simulink model "ModelForPicture"  (R2023a)
settings: Solver=VariableStepAuto  StartTime=0.0  StopTime=10.0  RelTol=1e-3
values from neighbouring files (symbols this model uses):
  timeStep = 0.005    [Cosim_Setup_SLC_MPC_T1_SP_LTR_Cosim_3D.m]
libraries: simulink x7, Solver_SF x1
settings Model: Creator=28303  LastModifiedBy=28303

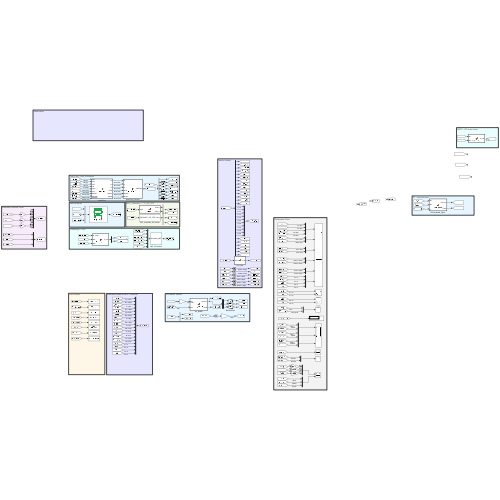
[thumbnail: Simulink's stored preview of the top-level diagram]
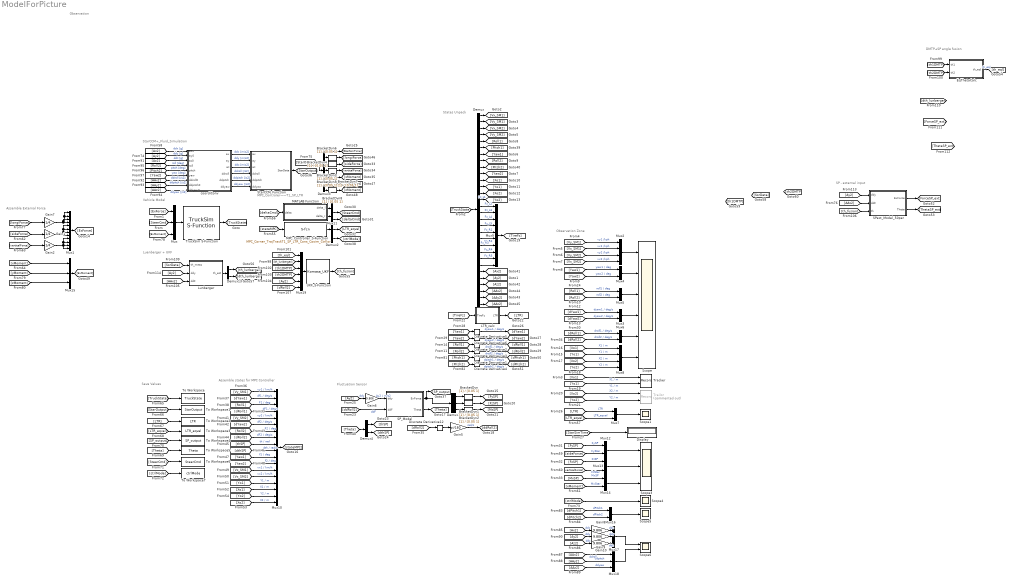
== system ModelForPicture ==
  note: Save Values
  note: StarCCM+_Fluid_Simulation
  note: Assemble states for MPC Controller
  note: Observation Zone
  note: Vehicle Model
  note: Fluctuation Sensor
  note: States Unpack
  note: Assemble External Force
  note: MPC_Controler——T1_SP_LTR
  note: Observation
  note: Luenberger + UKF
  note: SP - external input
  note: DMTP→SP angle fusion
  BracketDyn{,1..8} (9 alike) : TransferFcn  Denominator=[0.05 1]
  Demux : Demux  Outputs=30
  Demux1 : Demux  Outputs=3
  Demux13 : Demux  Outputs=2
  Demux2 : Demux  Outputs=3
  Demux3 : Demux  Outputs=7
  Demux4 : Demux  Outputs=2
  Discrete Derivative{1..6,12} (7 alike) : simulink/Discrete/Discrete Derivative  gainval=1.0  ICPrevScaledInput=0.0  OutMin=[]  OutMax=[]  OutDataType=fixdt(1, 16)  OutScaling=2^-10  DoSatur=off
  Display : Display
  EqThetaCalc : MATLAB Function  TreatAsAtomicUnit=on
  Gain1 : Gain  Gain=1/4
  Gain{6,8..10} (4 alike) : Gain  Gain=9.806
  Gain2 : Gain  Gain=1/4
  Gain5 : Gain  Gain=pi/180
  Gain7 : Gain  Gain=1/4
  "LTR_calc " : MATLAB Function  TreatAsAtomicUnit=on
  Lunberger : MATLAB Function  TreatAsAtomicUnit=on  SystemSampleTime=0.005
  MATLAB Function : MATLAB Function  TreatAsAtomicUnit=on
  MPC_Controller_S-Function : S-Function  FunctionName=MPC_Corner_TrajTrackT1_SP_LTR_Cons_Cosim_Ctrllor  SFunctionDeploymentMode=off  EnableBusSupport=off
  Mux{,15,17..18} (4 alike) : Mux  Inputs=3
  Mux1 : Mux  Inputs=12
  Mux10 : Mux  Inputs=18
  Mux{3..7,11..14,16} (10 alike) : Mux  Inputs=2
  Mux19 : Mux  Inputs=6
  Mux2 : Mux
  Mux8 : Mux
  Mux9 : Mux  Inputs=10
  SP_Model : MATLAB Function  TreatAsAtomicUnit=on  SystemSampleTime=0.005
  SPext_Model_50per : MATLAB Function  TreatAsAtomicUnit=on  SystemSampleTime=0.005
  Scope : Scope  NumInputPorts=6
  Scope1 : Scope
  Scope3 : Scope  NumInputPorts=3
  Scope4 : Scope
  Scope5 : Scope
  Scope6 : Scope  NumInputPorts=2
  StarCCM_Function : MATLAB Function  TreatAsAtomicUnit=on  SystemSampleTime=[timeStep 0]
  To Workspace : ToWorkspace  VariableName=TruckState  SaveFormat=Timeseries  SampleTime=-1
  To Workspace1 : ToWorkspace  VariableName=StarOutput  SaveFormat=Timeseries  SampleTime=-1
  To Workspace2 : ToWorkspace  VariableName=LTR  SaveFormat=Timeseries  SampleTime=-1
  To Workspace3 : ToWorkspace  VariableName=LTR_eqval  SaveFormat=Timeseries  SampleTime=-1
  To Workspace4 : ToWorkspace  VariableName=SP_output  SaveFormat=Timeseries  SampleTime=-1
  To Workspace5 : ToWorkspace  VariableName=Theta  SaveFormat=Timeseries  SampleTime=-1
  To Workspace6 : ToWorkspace  VariableName=SteerCmd  SaveFormat=Timeseries  SampleTime=-1
  To Workspace7 : ToWorkspace  VariableName=ctrlMode  SaveFormat=Timeseries  SampleTime=-1
  Tracker : Record  FileSettingsInternal="{\"entries\":[{\"content\":{\"excelSettings\":{\"content\":{},\"type\":\"Streamout.ExcelSettings\"}},\"type\":\"Streamout.FileSettingStorage\",\"uuid\":\"4a90c35d-7bfd-41ec-8da0-5aca52dec46b\"}],\"packageUris\":[\"http://schema.mathworks.com/mf0/streamout_blocks/R2020a\"],\"version\":\"1.0\"}"  Layout=[1 1]  SignalsInternal="{\"entries\":[{\"content\":{\"signals\":[{\"content\":{\"blockPath\":[\"ModelForPicture/Tracker\"],\"dimensions\":[1],\"domain\":\"ModelForPicture/Tracker\",\"lineColor\":\"#a2142f\",\"plots\":[1],\"port\":1,\"signalID\":60,\"signalName\":\"X1 / m\"},\"type\":\"RecordBlkView.Signal\",\"uuid\":\"e0ec3f2a-d673-4e95-a2c3-a892657a70bc\"},{\"content\":{\"blockPath\":[\"ModelForPicture/Tracker\"],\"dimensions\":[1],\"domain\":\"ModelForPicture/Tracker\",\"lineColor\":\"#139fff\",\"plots\":[1],\"port\":2,\"signalID\":63,\"signalName\":\"Y1 / m\"},\"type\":\"RecordBlkView.Signal\",\"uuid\":\"7fecea9c-d846-4e34-85a3-bedaa984d42a\"}]},\"type\":\"RecordBlkView.InputSignals\",\"uuid\":\"c903ce25-8e67-4217-b729-18382a9d9747\"}],\"packageUris\":[\"http://schema.mathworks.com/mf0/streamout_blocks/R2020a\"],\"version\":\"1.0\"}"  VisualizationBindings="{\"xyplotplugin\":{\"info\":[{\"series\":[{\"bindingParametersList\":[{\"parameter\":\"X-Axis\",\"signalID\":60,\"signalName\":\"X1 \\/ m\"},{\"parameter\":\"Y-Axis\",\"signalID\":63,\"signalName\":\"Y1 \\/ m\"}],\"seriesID\":59350}],\"subplotID\":1}]}}"  CompatibilityTag=XY  st=-1
  "Trailor " : Record  Commented=on  FileSettingsInternal="{\"entries\":[{\"content\":{\"excelSettings\":{\"content\":{},\"type\":\"Streamout.ExcelSettings\"}},\"type\":\"Streamout.FileSettingStorage\",\"uuid\":\"feb93b89-5eaa-4280-93fa-8b27e2285d0c\"}],\"packageUris\":[\"http://schema.mathworks.com/mf0/streamout_blocks/R2020a\"],\"version\":\"1.0\"}"  Layout=[1 1]  SignalsInternal="{\"entries\":[{\"content\":{\"signals\":[{\"content\":{\"blockPath\":[\"ModelForPicture/Trailor \"],\"dimensions\":[1],\"domain\":\"ModelForPicture/Trailor \",\"lineColor\":\"#a2142f\",\"plots\":[1],\"port\":1,\"signalID\":52,\"signalName\":\"XY Graph:1\"},\"type\":\"RecordBlkView.Signal\",\"uuid\":\"cce15bee-6aac-4d00-ab61-70a8d4efd641\"},{\"content\":{\"blockPath\":[\"ModelForPicture/Trailor \"],\"dimensions\":[1],\"domain\":\"ModelForPicture/Trailor \",\"lineColor\":\"#139fff\",\"plots\":[1],\"port\":2,\"signalID\":55,\"signalName\":\"XY Graph:2\"},\"type\":\"RecordBlkView.Signal\",\"uuid\":\"4f8b7c47-76ec-4c22-8b6d-3fa533720d48\"}]},\"type\":\"RecordBlkView.InputSignals\",\"uuid\":\"e5dfdc97-ae74-4c5b-8c00-5dfecc099489\"}],\"packageUris\":[\"http://schema.mathworks.com/mf0/streamout_blocks/R2020a\"],\"version\":\"1.0\"}"  VisualizationBindings="{\"xyplotplugin\":{\"info\":[{\"series\":[{\"bindingParametersList\":[{\"parameter\":\"X-Axis\",\"signalID\":52,\"signalName\":\"XY Graph:1\"},{\"parameter\":\"Y-Axis\",\"signalID\":55,\"signalName\":\"XY Graph:2\"}],\"seriesID\":41172}],\"subplotID\":1}]}}"  CompatibilityTag=XY  st=-1
  TruckSim S-Function : Solver_SF/TruckSim S-Function  Priority=1  SIMFILE=ALGO_Corner_Tanker_TrajTrack_MPC_T1_SP_LTR_Cosim_3D.sim
      settings: SourceProductName=TruckSim S-Function
  UKF_S-Function : S-Function  FunctionName=Komasa_UKF  SFunctionDeploymentMode=off  EnableBusSupport=off
  coordiConv : MATLAB Function  TreatAsAtomicUnit=on
  wires:
  Demux/23 -> Mux9/9  "Fz_R5"
  Demux2/3 -> [ctrlMode]
  [ctrlMode] -> To Workspace7/1
  [stateMPC] -> MPC_Controller_S-Function/1
  Demux/24 -> Mux9/10
  [Vx_SM2] -> Mux10/14  "vx2 / km/h"
  Mux12/1 -> Scope3/1
  [Yaw1] -> Mux10/11  "f1 / deg"
  [Vx_SM1] -> Mux10/13  "vx1 / km/h"
  BracketDyn5/1 -> [xMoment]
  [LTR] -> Mux7/1  "LTR"
  MATLAB Function/1(delta_l) -> Mux11/1
  [TruckState] -> Demux/1
  Mux13/1 -> Scope3/2
  [LTR_eqval] -> To Workspace3/1
  MPC_Controller_S-Function/1 -> Demux2/1
  Mux6/1 -> Scope/5
  [sideForce] -> Mux12/2  "FyStar"
  [Xo1] -> Mux10/16  "X1 / m"
  [TruckState] -> To Workspace/1
  [FySP] -> Mux12/1  "FySP"
  [thSP] -> Mux10/9  "th / rad"
  [verticalForce] -> Gain2/1
  [sideForce] -> Gain1/1
  Demux2/2 -> [LTR_eqval]
  Mux10/1 -> [stateMPC]
  [Roll1] -> Mux10/3  "F1 / deg"
  [SteerCmd] -> Mux/2
  [Yaw2] -> Mux4/2  "yaw2 / deg"
  [dRoll1] -> Mux10/4  "dF1 / deg/s"
  Mux9/1 -> [TireFz]
  [Xo1] -> Tracker/1  "X1 / m"
  [Yaw2] -> Discrete Derivative6/1
  [Xo2] -> "Trailor "/1  "X2 / m"
  [Xo2] -> Mux8/3  "X2 / m"
  [Roll2] -> Discrete Derivative3/1
  Mux4/1 -> Scope/2
  [dthSP] -> Mux10/10  "dth / rad/s"
  Discrete Derivative2/1 -> [dRoll1]  "droll1 / deg/s"
  Demux2/1 -> [deltaCmd]
  Discrete Derivative5/1 -> [dYaw1]  "dyaw1 / deg/s"
  "LTR_calc "/1(LTR) -> [LTR]
  [Roll1] -> Discrete Derivative2/1
  [Yaw1] -> Mux4/1  "yaw1 / deg"
  [Vx_SM1] -> Mux2/2  "vx1 /kph"
  Mux1/1 -> [ExForce]
  [Yo2] -> "Trailor "/2  "Y2 / m"
  Demux1/1 -> BracketDyn/1
  Mux/1 -> TruckSim S-Function/1
  Mux2/1 -> Scope/1
  [Yo1] -> Mux8/2  "Y1 / m"
  [Vy_SM2] -> Mux2/3  "vy2 /kph"
  [Roll2] -> Mux5/2  "roll2 / deg"
  SP_Model/2(Theta) -> [Theta]
  [Yo1] -> Tracker/2  "Y1 / m"
  [ExForce] -> Mux/1
  SP_Model/1(ExForce) -> [SP_output], Demux1/1
  Gain2/1 -> Mux1/9, Mux1/10, Mux1/12, Mux1/11
  Discrete Derivative12/1 -> Gain5/1
  Gain6/1 -> SP_Model/1(ddy)  "Ay2 / m/s2"
  [dYaw1] -> Mux3/1  "dyaw1 / deg/s"
  [dRoll2] -> Mux10/8  "dF2 / deg/s"
  [dRoll2] -> Discrete Derivative12/1
  Demux4/2 -> [dthSP]
  Demux/18 -> Mux9/4  "Fz_L5"
  Demux/20 -> Mux9/6  "Fz_R2"
  Demux/26 -> [Ay2]
  Mux7/1 -> Scope1/1
  Demux/7 -> [Yaw1]
  Demux/6 -> [Pitch1]
  BracketDyn/1 -> [FySP]
  Demux/15 -> Mux9/1  "Fz_L2"
  [StarOutput] -> Demux3/1
  Demux/14 -> [Yo2]  "Fz_L1"
  Demux/27 -> [Az2]
  [Vx_SM2] -> Mux2/4  "vx2 /kph"
  [xMoment] -> Mux15/1
  [Vy_SM1] -> Mux2/1  "vy1 /kph"
  Mux11/1 -> [SteerCmd]
  [Theta] -> To Workspace5/1
  [Ay2] -> Gain6/1  "ddy"
  [AAx2] -> coordiConv/7(ddroll0)  "ddroll [/s2]"
  [Pitch2] -> coordiConv/5(pitch)  "pitch [deg]"
  Demux3/6 -> BracketDyn7/1
  Demux/4 -> [Vy_SM2]
  coordiConv/2(ay) -> StarCCM_Function/2(ay)  "ddy [m/s2]"
  [dYaw1] -> Mux10/2  "df1 / deg/s"
  Demux3/1 -> [StarSimTime]
  [LTR_eqval] -> Mux7/2  "LTR_eqval"
  BracketDyn7/1 -> [yMoment]
  [Roll1] -> Mux5/1  "roll1 / deg"
  [yMoment] -> Mux15/2
  Demux/12 -> [Yo1]
  [Yo1] -> Mux10/15  "Y1 / m"
  Demux/19 -> Mux9/5  "Fz_R1"
  Demux/16 -> Mux9/2  "Fz_L3"
  [xMoment] -> Mux14/2  "MxStar"
  Demux/3 -> [Vx_SM2]
  Discrete Derivative3/1 -> [dRoll2]  "droll2 / deg/s"
  TruckSim S-Function/1 -> [TruckState]
  coordiConv/4(ddroll) -> StarCCM_Function/4(ddroll)  "ddroll [/s2]"
  [Theta] -> Demux4/1
  [ddRoll2] -> SP_Model/2(ddF)  "ddF"
  [Roll2] -> Mux10/7  "F2 / deg"
  coordiConv/5(ddpitch) -> StarCCM_Function/5(ddpitch)  "ddpitch [/s2]"
  [Yo2] -> Mux10/17  "Y2 / m"
  Mux14/1 -> Scope3/3
  coordiConv/6(ddyaw) -> StarCCM_Function/6(ddyaw)  "ddyaw [/s2]"
  [Az2] -> coordiConv/3(az0)  "ddz [g]"
  coordiConv/3(az) -> StarCCM_Function/3(az)  "ddz [m/s2]"
  [Roll2] -> coordiConv/4(roll)  "roll [deg]"
  Mux3/1 -> Scope/4
  coordiConv/1(ax) -> StarCCM_Function/1(ax)  "ddx [m/s2]"
  [Xo2] -> Mux10/18  "X2 / m"
  [AAz2] -> coordiConv/9(ddyaw0)  "ddyaw [/s2]"
  [AAy2] -> coordiConv/8(ddpitch0)  "ddpitch [/s2]"
  Mux8/1 -> Scope/6
  [dYaw2] -> Mux10/6  "df2 / deg/s"
  Mux17/1 -> Scope6/1
  [SteerCmd] -> To Workspace6/1
  [Vy_SM2] -> Mux10/5  "vy2 / km/h"
  [FzSP] -> Mux13/1  "FzSP"
  Mux15/1 -> [ExMoment]
  Mux16/1 -> Scope5/1
  MATLAB Function/2(delta_r) -> Mux11/2
  [StarOutput] -> To Workspace1/1
  Demux1/3 -> BracketDyn2/1
  BracketDyn6/1 -> [longiForce]
  Demux1/2 -> BracketDyn1/1
  Mux5/1 -> Scope/3
  Demux/5 -> [Roll1]
  [Ax2] -> coordiConv/1(ax0)  "ddx [g]"
  Demux/13 -> [Xo2]
  [Yaw1] -> Discrete Derivative5/1
  Discrete Derivative4/1 -> [dPitch2]  "dpitch2 / deg/s"
  Discrete Derivative1/1 -> [dPitch1]  "dpitch1 / deg/s"
  [Vy_SM1] -> Mux10/1  "vy1 / km/h"
  BracketDyn1/1 -> [FzSP]
  [AAz2] -> Mux18/3  "ddyaw"
  [Ax2] -> Gain8/1  "ddx"
  [zMoment] -> Mux15/3
  BracketDyn2/1 -> [MxSP]
  Demux/28 -> [AAx2]
  [Xo1] -> Mux8/1  "X1 / m"
  [AAy2] -> Mux18/2  "ddpitch"
  Gain8/1 -> Mux17/1  "ddx"
  [Ay2] -> Gain9/1  "ddy"
  Demux4/1 -> [thSP]
  BracketDyn4/1 -> [sideForce]
  [Az2] -> Gain10/1  "ddz"
  Demux3/7 -> BracketDyn8/1
  [TireFz] -> "LTR_calc "/1(TireFz)
  [Pitch2] -> Discrete Derivative4/1
  [StarSimTime] -> Display/1
  [Yaw2] -> coordiConv/6(yaw)  "yaw [deg]"
  [ExMoment] -> Mux/3
  Mux18/1 -> Scope6/2
  Demux/25 -> [Ax2]
  Demux/8 -> [Roll2]
  [AAx2] -> Mux18/1  "ddroll"
  [dRoll2] -> Mux6/2  "droll2 / deg/s"
  Demux3/4 -> BracketDyn3/1
  Demux3/3 -> BracketDyn4/1
  [Pitch1] -> Discrete Derivative1/1
  [LTR] -> To Workspace2/1
  Demux/9 -> [Pitch2]
  Gain9/1 -> Mux17/2  "ddy"
  [dPitch1] -> Mux16/1  "dPitch1"
  Demux3/5 -> BracketDyn5/1
  [dPitch2] -> Mux16/2  "dPitch2"
  StarCCM_Function/1(StarData) -> [StarOutput]
  [SP_output] -> To Workspace4/1
  BracketDyn3/1 -> [verticalForce]
  [Ay2] -> coordiConv/2(ay0)  "ddy [g]"
  Discrete Derivative6/1 -> [dYaw2]  "dyaw2 / deg/s"
  Demux/11 -> [Xo1]
  [longiForce] -> Gain7/1
  Demux/2 -> [Vy_SM1]
  BracketDyn8/1 -> [zMoment]
  [MxSP] -> Mux14/1  "MxSP"
  Gain7/1 -> Mux1/3, Mux1/1, Mux1/2, Mux1/4
  [verticalForce] -> Mux13/2  "FzStar"
  [ctrlMode] -> Scope4/1
  [dRoll1] -> Mux6/1  "droll1 / deg/s"
  Gain5/1 -> [ddRoll2]  "rad/s"
  Demux/29 -> [AAy2]
  Demux/1 -> [Vx_SM1]
  Demux3/2 -> BracketDyn6/1
  Demux/22 -> Mux9/8  "Fz_R4"
  [dYaw2] -> Mux3/2  "dyaw2 / deg/s"
  [Yo2] -> Mux8/4  "Y2 / m"
  Gain10/1 -> Mux17/3  "ddz"
  Demux/17 -> Mux9/3  "Fz_L4"
  Demux/21 -> Mux9/7  "Fz_R3"
  Gain1/1 -> Mux1/8, Mux1/6, Mux1/5, Mux1/7
  [Yaw2] -> Mux10/12  "f2 / deg"
  Demux/30 -> [AAz2]
  Demux/10 -> [Yaw2]
  [deltaCmd] -> MATLAB Function/1(delta)
  Demux13/1 -> [th_lunberger]
  SPext_Model_50per/1(ExForce) -> [ForceSP_ext]
  [th_lunberger] -> Mux19/2
  [th1DMTP] -> EqThetaCalc/1(th1)
  [SsrData] -> Lunberger/1(th_meas)
  [Ay2] -> Lunberger/2(ddy)
  UKF_S-Function/1 -> [th_fusion]
  Lunberger/1(th_est) -> Demux13/1
  [AAx2] -> Lunberger/3(ddF)
  Demux13/2 -> [dth_lunberger]
  [th_fusion] -> SPext_Model_50per/3(th)
  [Ay2] -> Mux19/5
  [dRoll2] -> Mux19/6
  [th2DMTP] -> EqThetaCalc/2(th2)
  [th2DMTP] -> Mux19/4
  Mux19/1 -> UKF_S-Function/1
  [th1DMTP] -> Mux19/3
  EqThetaCalc/1(th_eql) -> [th_eql]  "th_eql"
  SPext_Model_50per/2(Theta) -> [ThetaSP_ext]
  [th_eql] -> Mux19/1
  [Ay2] -> SPext_Model_50per/1(ddy)
  [AAx2] -> SPext_Model_50per/2(ddF)

== matlab function ModelForPicture/SP_Model ==
  data: ddy input; ExForce output; ddF input; Theta output
function [ExForce,Theta] = SP_Model(ddy,ddF)
persistent sim_param Ts y0
%% 定义摆
if isempty(Ts)
%SP模型，共5个参数拟合
% 参数 m1 h0 hp lp coeff
x=[10890,1.5,0.13,0.97,0.13];
% 获取参数
sim_param=getParam_SP(x);
%初始状态量
y0=zeros(9,1);
%采样时间
Ts=0.005;
end

y=y0;

%% 求解微分方程
dy=zeros(9,1);
dy(1)=y(2);
dy(2)=ddy;
dy(3)=(dy(2)-y(3))/Ts;
dy(4)=y(5);
dy(5)=ddF;
dy(6)=(dy(5)-y(6))/Ts;
dy(7)=y(8);
dy(8)=calc_ddth_SP(y,sim_param);
dy(9)=(dy(8)-y(9))/Ts;
y=y0+dy*Ts;
%% 计算三向力输出
[Fy,Fz,Mx]=calc_Fp_SP(y,sim_param);
ExForce=[Fy,Fz,Mx];
%% 更新状态量
y0=y;
th=y(7);
dth=y(8);
Theta=[th,dth];
end

%% 根据变量获取参数
function sim_param=getParam_SP(x)
%根据变量生成传输参数
TotMass=14462;
m1=x(1);%参数1
m0=TotMass-m1;
h0=x(2);%参数2
hp=x(3);%参数3
lp=x(4);%参数4
g=9.806;
coeff=x(5);%参数5
sim_param=[m0,m1,h0,hp,lp,g,coeff];
end

%% 求解三向力输出
function [Fy,Fz,Mx] = calc_Fp_SP(state,param)
% sim_param=[m0,m1,h0,hp,lp,g,coeff];
m0=param(1);
m1=param(2);
h0=param(3);
hp=param(4);
lp=param(5);
g=param(6);
% co=param(7);

% y=state(1);
% dy=state(2);
ddy=state(3);
f=state(4);
df=state(5);
ddf=state(6);
th=state(7);
dth=state(8);
ddth=state(9);

%定义运算符简写
sf=sin(f);
cf=cos(f);
s2=sin(th+f);
c2=cos(th+f);
L=lp+hp;
%定义质量块的 位置矢量
exh=0.77; %额外增加的高度是罐底到车轴心的高度
R0=[-(exh+h0)*sf,(exh+h0)*cf];

R1=[-(exh+L)*sf+lp*s2
    (exh+L)*cf-lp*c2];

ddRp0=[ddy-h0*cf*ddf+df^2*h0*sf
-h0*sf*ddf-h0*cf*df^2+g];

ddRp1=[ddy+ddf*(-L*cf+lp*c2)+ddth*(lp*c2)+df^2*(L*sf-lp*s2)+dth^2*(-lp*s2)+df*dth*(-2*lp*s2)
ddf*(-L*sf+lp*s2)+ddth*(lp*s2)+df^2*(-L*cf+lp*c2)+dth^2*(lp*c2)+df*dth*(2*lp*c2)+g];

Fp=m0*ddRp0+m1*ddRp1;
Fy=Fp(1)*cf-(-Fp(2))*sf;
Fz=(-Fp(2))*cf+Fp(1)*sf;
Mx0=(m0*(R0(1)*-ddRp0(2)+R0(2)*ddRp0(1)));
Mx1=(m1*(R1(1)*-ddRp1(2)+R1(2)*ddRp1(1)));

Mx=Mx0+Mx1;

end
%% 求解ddth
function ddth = calc_ddth_SP(state,param)
% sim_param=[m0,m1,h0,hp,lp,g,coeff];
% m0=param(1);
% m1=param(2);
% h0=param(3);
hp=param(4);
lp=param(5);
g=param(6);
co=param(7);

% y=state(1);
% dy=state(2);
ddy=state(3);
f=state(4);
df=state(5);
ddf=state(6);
th=state(7);
dth=state(8);
% ddth=state(9);


%定义运算符简写
s1=sin(th);
c1=cos(th);
s2=sin(th+f);
c2=cos(th+f);
L=lp+hp;

ddth=-(ddy*lp*c2+ddf*(-lp*L*c1+lp^2)-df^2*lp*L*s1+g*lp*s2)/(lp^2);
ddth=ddth-co*dth;

end

== matlab function ModelForPicture/LTR_calc  ==
  data: TireFz input; LTR output
function LTR = fcn(TireFz)
% 分配物理量
FzL=sum(TireFz(1:5));
FzR=sum(TireFz(6:10));
% 进行计算
LTR=(FzL-FzR)/(FzL+FzR);
end

== matlab function ModelForPicture/StarCCM_Function ==
  data: ax input; StarData output; ay input; az input; ddroll input; ddpitch input; ddyaw input
function StarData = StarCCM_Fun(ax,ay,az,ddroll,ddpitch,ddyaw)
%定义标志位路径
java_flag = 'java_flag.csv';
matlab_flag = 'matlab_flag.csv';
%定义输出文件路径
java_output = 'java_output.csv';
matlab_output = 'matlab_output.csv';

%状态1：从StarCCM+的输出文件中提取数据

DataConv=getLastLineNum(java_output);
StarData=DataConv(1:7);

%状态2：Simulink利用获得的数据进行下一个仿真步

%状态3：Simulink输出数据文件，暂停自身的仿真
Matlab_Data=[ax,ay,az,ddroll,ddpitch,ddyaw];
writeData(Matlab_Data,matlab_output);

%状态4：置位matlab_flag标志位，允许StarCCM+采集数据
setFlag(matlab_flag);

%状态5：不断检测java_flag标志位，等待StarCCM+仿真结束
while(~getFlag(java_flag))
end
resetFlag(java_flag)
%进入下一个循环，回到状态1

end
%*************函数writeData*****************
%参数：data，数值向量
%参数：dir,目标输出文件地址
%将data转换为精度30的字符串写入目标文件
%*****************************************
function writeData(data,dir)
len=length(data);
buffer=sprintf('%0.10f',data(1));
if(len>=2)
    for i=2:len
    buffer=[buffer ',' sprintf('%0.10f',data(i))];
    end
    str=buffer;
else
    str='';
end

fileID = fopen(dir,'w');
fwrite(fileID,str,'char');
fclose(fileID);

end

%*************函数getLastLineNum*****************
%参数：dir,标志位文件的路径
%返回值：data,获得数据文件的最后一行并转换为数字数组
%*****************************************
function data=getLastLineNum(dir)
str=readLastLine(dir);
data=stringSplit(str,',');
end

%*************函数stringSplit*****************
%参数：str,待分割的字符串
%参数：notion,字符，用于指定分割的字符
%返回值：data,字符串数组，将字符串按照指定方式分割
%*****************************************
function data=stringSplit(str,notion)
len=length(str);
splitPlace=0;
for i=1:len
if(str(i)==notion)
splitPlace=[splitPlace i];

end
end
splitNum=length(splitPlace);
splitPlace=[splitPlace len+1];

data=zeros(1,splitNum);
for i=1:splitNum
data(i)=real(str2double(str((splitPlace(i)+1):(splitPlace(i+1)-1))));
end

end
%*************函数readLastLine*****************
%参数：dir,标志位文件的路径
%返回值：lastLine,字符串，最后一行的内容
%*****************************************
function lastLine=readLastLine(dir)
fileID = fopen(dir,'r');     %# Open the file as a binary
lastLine = '';                   %# Initialize to empty
offset = 1;                      %# Offset from the end of file
fseek(fileID,-offset,'eof');        %# Seek to the file end, minus the offset
newChar = fread(fileID,1,'char');  %# Read one character
while (newChar~=10) | (offset == 1)
  lastLine = [newChar lastLine];   %# Add the character to a string
  offset = offset+1;
  fseek(fileID,-offset,'eof');        %# Seek to the file end, minus the offset
  newChar = fread(fileID,1,'char');  %# Read one character
end
fclose(fileID);  %# Close the file
end
%*************函数getFlag*****************
%参数：dir,标志位文件的路径
%返回值：flag,获得标志位文件的内容，返回一个字节
%标志位,文件内容为'1'(49)则flag为1
%文件内容为'0'(48)则flag为0（其他非'1'内容则flag也为0）
%*****************************************
function flag=getFlag(dir)
fileID = fopen(dir,'r');%,'n','UTF-8'
    A = fread(fileID,1,'char');
    if(A==49)
    flag=1;
    else 
    flag=0;
    end
fclose(fileID);
end
%*************函数setFlag*****************
%参数：dir,标志位文件的路径
%返回值：无
%作用：重置标志位文件内容为'1'(49)
%*****************************************
function setFlag(dir)
fileID = fopen(dir,'w');
fwrite(fileID,'1','char');
fclose(fileID);
end
%*************函数resetFlag*****************
%参数：dir,标志位文件的路径
%返回值：无
%作用：重置标志位文件内容为'0'(48)
%*****************************************
function resetFlag(dir)
fileID = fopen(dir,'w');
fwrite(fileID,'0','char');
fclose(fileID);
end

== matlab function ModelForPicture/coordiConv ==
  data: ax0 input; ax output; ay0 input; az0 input; roll input; pitch input; yaw input; ddroll0 input; ddpitch0 input; ddyaw0 input; ay output; az output; ddroll output; ddpitch output; ddyaw output
function [ax,ay,az,ddroll,ddpitch,ddyaw]= coordiConv(ax0,ay0,az0,roll, pitch, yaw,ddroll0,ddpitch0,ddyaw0)%输入的旋转是角度degree
persistent g
if isempty(g)
    g = 9.806;
end

vec = Rotation3D([0;0;g], roll, pitch, yaw);


ax = -(vec(1) + ax0*g);
ay = -(vec(2) + ay0*g);
az = -(vec(3) + az0*g);

ddroll = -ddroll0;
ddpitch = -ddpitch0;
ddyaw = -ddyaw0;

end


function vec = Rotation3D(vec0, roll, pitch, yaw)
    % 将角度从度转换为弧度
    roll = deg2rad(roll);
    pitch = deg2rad(pitch);
    yaw = deg2rad(yaw);

    % 创建绕x轴旋转的旋转矩阵（Roll）
    Rx = [1, 0, 0;
          0, cos(roll), -sin(roll);
          0, sin(roll), cos(roll)];

    % 创建绕y轴旋转的旋转矩阵（Pitch）
    Ry = [cos(pitch), 0, sin(pitch);
          0, 1, 0;
          -sin(pitch), 0, cos(pitch)];

    % 创建绕z轴旋转的旋转矩阵（Yaw）
    Rz = [cos(yaw), -sin(yaw), 0;
          sin(yaw), cos(yaw), 0;
          0, 0, 1];

    % 综合旋转矩阵
    R = Rz * Ry * Rx;

    % 应用旋转矩阵到向量
    vec = R * vec0;
end

== matlab function ModelForPicture/MATLAB Function ==
  data: delta input; delta_l output; delta_r output
function [delta_l, delta_r] = Ackerman(delta)

delta_l = delta*180/pi;
delta_r = delta*180/pi;

== matlab function ModelForPicture/EqThetaCalc ==
  data: th1 input; th_eql output; th2 input
function th_eql = EqThetaCalc(th1,th2)
persistent l k r m1 m2
if isempty(l)
    m1=6.9390e+03;
    m2=3.0429e+03;
    k=10*m2/(m1+m2);
    l=0.432;
    r=0.579;
end
% th_eql=atan((l*sin(th1)+k*r*sin(th1+th2))/...
%             (l*cos(th1)+k*r*cos(th1+th2)));
%  th_eql=(th1*m1+th2*m2)/(m1+m2);
  th_eql=(th1*(m1+m2)+th2*m2)/(m1+m2+m2);

end

== matlab function ModelForPicture/SPext_Model_50per ==
  data: ddy input; ExForce output; ddF input; Theta output; th input
function [ExForce,Theta] = SPext_Model(ddy,ddF,th)
persistent sim_param Ts y0 th0 dth0
%% 定义摆
if isempty(Ts)
%SP模型，共5个参数拟合
% 参数 m1 h0 hp lp coeff
x=[10890,1.5,0.13,0.97,0.13];
% 获取参数
sim_param=getParam_SP(x);
%初始状态量
y0=zeros(9,1);
th0=0;
dth0=0;
%采样时间
Ts=0.005;
end

y=y0;

%% 求解微分方程
dy=zeros(9,1);
dy(1)=y(2);
dy(2)=ddy;
dy(3)=(dy(2)-y(3))/Ts;
dy(4)=y(5);
dy(5)=ddF;
dy(6)=(dy(5)-y(6))/Ts;
dy(7)=y(8);
dy(8)=calc_ddth_SP(y,sim_param);
dy(9)=(dy(8)-y(9))/Ts;
y=y0+dy*Ts;
y(7)=th;
dth=(th-th0)/Ts;
y(8)=dth;
y(9)=(dth-dth0)/Ts;
th0=th;
dth0=dth;
%% 计算三向力输出
[Fy,Fz,Mx]=calc_Fp_SP(y,sim_param);
ExForce=[Fy,Fz,Mx];
%% 更新状态量
y0=y;
th=y(7);
dth=y(8);
Theta=[th,dth];
end

%% 根据变量获取参数
function sim_param=getParam_SP(x)
%根据变量生成传输参数
TotMass=14462;
m1=x(1);%参数1
m0=TotMass-m1;
h0=x(2);%参数2
hp=x(3);%参数3
lp=x(4);%参数4
g=9.806;
coeff=x(5);%参数5
sim_param=[m0,m1,h0,hp,lp,g,coeff];
end

%% 求解三向力输出
function [Fy,Fz,Mx] = calc_Fp_SP(state,param)
% sim_param=[m0,m1,h0,hp,lp,g,coeff];
m0=param(1);
m1=param(2);
h0=param(3);
hp=param(4);
lp=param(5);
g=param(6);
% co=param(7);

% y=state(1);
% dy=state(2);
ddy=state(3);
f=state(4);
df=state(5);
ddf=state(6);
th=state(7);
dth=state(8);
ddth=state(9);

%定义运算符简写
sf=sin(f);
cf=cos(f);
s2=sin(th+f);
c2=cos(th+f);
L=lp+hp;
%定义质量块的 位置矢量
exh=0.77; %额外增加的高度是罐底到力矩受力中心车轴中心的高度
R0=[-(h0+exh)*sf,(exh+h0)*cf];

R1=[-(L+exh)*sf+lp*s2
    (L+exh)*cf-lp*c2];

ddRp0=[ddy-h0*cf*ddf+df^2*h0*sf
-h0*sf*ddf-h0*cf*df^2+g];

ddRp1=[ddy+ddf*(-L*cf+lp*c2)+ddth*(lp*c2)+df^2*(L*sf-lp*s2)+dth^2*(-lp*s2)+df*dth*(-2*lp*s2)
ddf*(-L*sf+lp*s2)+ddth*(lp*s2)+df^2*(-L*cf+lp*c2)+dth^2*(lp*c2)+df*dth*(2*lp*c2)+g];

Fp=m0*ddRp0+m1*ddRp1;
Fy=Fp(1)*cf-(-Fp(2))*sf;
Fz=(-Fp(2))*cf+Fp(1)*sf;
Mx0=(m0*(R0(1)*-ddRp0(2)+R0(2)*ddRp0(1)));
Mx1=(m1*(R1(1)*-ddRp1(2)+R1(2)*ddRp1(1)));

Mx=Mx0+Mx1;

end
%% 求解ddth
function ddth = calc_ddth_SP(state,param)
% sim_param=[m0,m1,h0,hp,lp,g,coeff];
% m0=param(1);
% m1=param(2);
% h0=param(3);
hp=param(4);
lp=param(5);
g=param(6);
co=param(7);

% y=state(1);
% dy=state(2);
ddy=state(3);
f=state(4);
df=state(5);
ddf=state(6);
th=state(7);
dth=state(8);
% ddth=state(9);


%定义运算符简写
s1=sin(th);
c1=cos(th);
s2=sin(th+f);
c2=cos(th+f);
L=lp+hp;

ddth=-(ddy*lp*c2+ddf*(-lp*L*c1+lp^2)-df^2*lp*L*s1+g*lp*s2)/(lp^2);
ddth=ddth-co*dth;

end

== matlab function ModelForPicture/Lunberger ==
  data: th_meas input; th_est output size=[2 1]; ddy input; ddF input
function th_est = Luenberger(th_meas,ddy,ddF)
persistent A B C Ts xk_1
if isempty(Ts)
    Ts=0.005;
    g=9.806;
    hp=0.13;
    lp=0.97;
    c=0.13;
    A=[0  1;-g/lp -c];
    B=[0 0;1/lp hp/lp];
    C=[1 0];
    xk_1=[0 0]';
end
coder.extrinsic('luenbergerObserver');
L0 = luenbergerObserver(A,C,[-5,-5]);
L=zeros(2,1);
L(1:2,1)=L0(1:2,1);
[Ad,Bd] = c2d_zoh((A-L*C),[B,L],Ts);
xk=Ad*xk_1+Bd*[-ddy,ddF,th_meas]';
% th_est=C*xk;
th_est=xk;
xk_1=xk;
end
